simulink model "sample02_speed1"  (R2023a)
settings: Solver=ode1  StartTime=0.0  StopTime=inf  FixedStep=0.005  RelTol=1e-3  EnableMultiTasking=on
libraries: arduinolib x7, simulink x2
settings Model: ExtModeTrigDuration=2  Creator=kawata  LastModifiedBy=kawata
settings SolverCC: AutoInsertRateTranBlk=on
settings DataIOCC: ReturnWorkspaceOutputs=off
settings OptimizationCC: EnhancedBackFolding=on  PassReuseOutputArgsAs=Individual arguments  ZeroExternalMemoryAtStartup=off  ZeroInternalMemoryAtStartup=off  MaxStackSize=64  OptimizeBlockOrder=speed  DifferentSizesBufferReuse=on  OptimizationCustomize=off  EfficientTunableParamExpr=on
settings DebuggingCC: ParameterTunabilityLossMsg=error
settings HardwareCC: ProdBitPerInt=16  ProdBitPerPointer=16  ProdBitPerSizeT=16  ProdBitPerPtrDiffT=16  ProdLargestAtomicFloat=None  ProdWordSize=8  ProdHWDeviceType=Atmel->AVR  UseEmbeddedCoderFeatures=off  UseSimulinkCoderFeatures=off
settings SFSimCC: MATLABDynamicMemAlloc=off
settings RTWCC: Description=Embedded Coder  SystemTargetFile=ert.tlc  HardwareBoard=Arduino Mega 2560  TemplateMakefile=ert_default_tmf  Toolchain=Arduino AVR  BuildConfiguration=Faster Runs  GPUComputeCapability=5.0
settings CodeAppCC: ForceParamTrailComments=on  IgnoreCustomStorageClasses=off  OperatorAnnotations=on  SimulinkDataObjDesc=on  SFDataObjDesc=on  InsertBlockDesc=on
settings ERTTargetCC: SupportContinuousTime=on  SupportNonInlinedSFcns=on  SupportVariableSizeSignals=on  ExtModeTransport=3  ExtModeStaticAlloc=on  ExtModeAutomaticAllocSize=off  ExtModeStaticAllocSize=2048  ExtModeMexFile=ext_xcp  ExtModeIntrfLevel=Level2 - Open

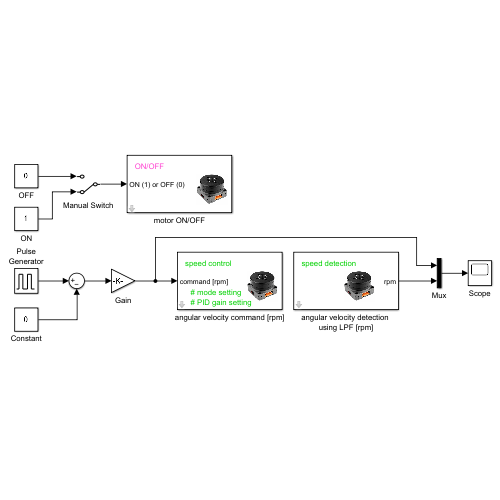
[thumbnail: Simulink's stored preview of the top-level diagram]
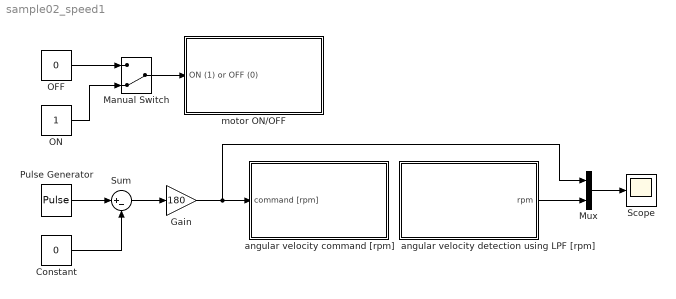
== system sample02_speed1 ==
  Constant : Constant  Value=0
  Gain : Gain  Gain=180
  Manual Switch : ManualSwitch  CurrentSetting=0
  Mux : Mux  Inputs=2
  OFF : Constant  Value=0
  ON : Constant
  Pulse Generator : DiscretePulseGenerator  PulseType=Time based  Period=4  PulseWidth=50  PhaseDelay=1
  Scope : Scope
  Sum : Sum  Inputs=|+-
  angular velocity command [rpm] : Subsystem  mask(angular velocity command [rpm]){I2CAddress=0x64, set_time=0, speed_P=15, speed_I=0.0001, speed_D=400}
      mask prompts: I2CAddress "I2C Address"; set_time "Set Time"; speed_P "P"; speed_I "I"; speed_D "D"
      mask help:
      | speed mode
      | ---------------------------------
      | default value (PID gain of speed controller)
      |  P: 15
      |  I: 0.0001
      |  D: 400
      | ---------------------------------
      | If t ≤ set_time, then PID gain can be set.
      mask DialogControl ParameterGroupVar Prompt: パラメーター
      mask Display:
      | image('roller485.png', [55,10,75,56]);
      | color('green');
      | text(10, 60, 'speed control');
      | text(17, 22, '# mode setting');
      | text(17, 10, '# PID gain setting');
  angular velocity detection using LPF [rpm] : Subsystem  mask{I2CAddress=0x64, sample_time=0.005}
      mask prompts: I2CAddress "I2C Address"; sample_time "Sample Time"
      mask DialogControl ParameterGroupVar Prompt: パラメーター
      mask Display:
      | image('roller485.png', [30,10,75,56]);
      | color('green');
      | text(10, 60, 'speed detection');
  motor ON/OFF : Subsystem  mask{I2CAddress=0x64}
      mask prompts: I2CAddress "I2C Address"
      mask help:
      | 0: motor off
      | 1: motor on
      mask DialogControl ParameterGroupVar Prompt: パラメーター
      mask Display:
      | image('roller485.png', [55,10,75,56]);
      | color('magenta');
      | text(10, 60, 'ON/OFF');
  wires:
  Manual Switch/1 -> motor ON/OFF/1(ON (1) or OFF (0))
  OFF/1 -> Manual Switch/1
  ON/1 -> Manual Switch/2
  Gain/1 -> angular velocity command [rpm]/1(command [rpm]), Mux/1
  Sum/1 -> Gain/1
  Constant/1 -> Sum/2
  Pulse Generator/1 -> Sum/1
  angular velocity detection using LPF [rpm]/1(rpm) -> Mux/2
  Mux/1 -> Scope/1

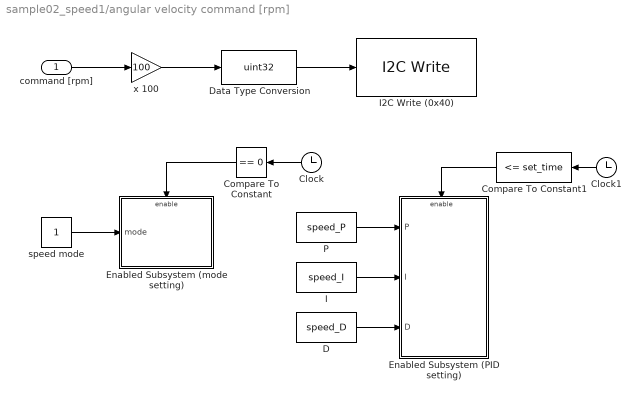
== system sample02_speed1/angular velocity command [rpm] ==
  command [rpm] : Inport
  "Clock " : Clock
  Clock1 : Clock
  Compare To Constant : simulink/Logic and Bit Operations/Compare To Constant  relop===  const=0  OutDataTypeStr=boolean
  Compare To Constant1 : simulink/Logic and Bit Operations/Compare To Constant  relop=<=  const=set_time  OutDataTypeStr=boolean
  D : Constant  Value=speed_D
  Data Type Conversion : DataTypeConversion  OutDataTypeStr=uint32  SaturateOnIntegerOverflow=off  RndMeth=Floor
  Enabled Subsystem (PID setting) : Subsystem  TreatAsAtomicUnit=on
  Enabled Subsystem (mode setting) : Subsystem  TreatAsAtomicUnit=on
  I : Constant  Value=speed_I
  I2C Write (0x40) : arduinolib/I2C Write  I2CModule=0  Mode=Master  SlaveAddress=I2CAddress  SlaveByteOrder=LittleEndian  Direction=Transmitter  RegisterAddressMode=on  RegisterAddress=0x40  SlaveDataType=uint8  DataLength=1  NoAck=off  RepeatedStart=off  OutputStatus=off  blockPlatform=ARDUINO
  P : Constant  Value=speed_P
  speed mode : Constant
  x 100 : Gain  Gain=100
  wires:
  x 100/1 -> Data Type Conversion/1
  command [rpm]/1 -> x 100/1
  Data Type Conversion/1 -> I2C Write (0x40)/1
  I/1 -> Enabled Subsystem (PID setting)/2(I)
  Clock1/1 -> Compare To Constant1/1
  P/1 -> Enabled Subsystem (PID setting)/1(P)
  speed mode/1 -> Enabled Subsystem (mode setting)/1(mode)
  Compare To Constant1/1 -> Enabled Subsystem (PID setting)/Enable
  Compare To Constant/1 -> Enabled Subsystem (mode setting)/Enable
  "Clock "/1 -> Compare To Constant/1
  D/1 -> Enabled Subsystem (PID setting)/3(D)

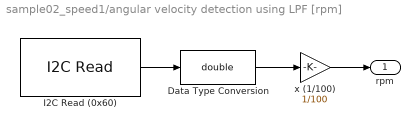
== system sample02_speed1/angular velocity detection using LPF [rpm] ==
  Data Type Conversion : DataTypeConversion  OutDataTypeStr=double  SaturateOnIntegerOverflow=off  RndMeth=Floor
  I2C Read (0x60) : arduinolib/I2C Read  I2CModule=0  Mode=Master  SlaveAddress=0x64  SlaveByteOrder=LittleEndian  Direction=Receiver  RegisterAddressMode=on  RegisterAddress=0x60  SlaveDataType=int32  DataLength=1  NoAck=off  RepeatedStart=off  OutputStatus=off  blockPlatform=ARDUINO  SampleTime=sample_time
  x (1/100) : Gain  Gain=1/100
  rpm : Outport
  wires:
  I2C Read (0x60)/1 -> Data Type Conversion/1
  Data Type Conversion/1 -> x (1/100)/1
  x (1/100)/1 -> rpm/1

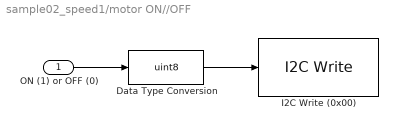
== system sample02_speed1/motor ON//OFF ==
  ON (1) or OFF (0) : Inport
  Data Type Conversion : DataTypeConversion  OutDataTypeStr=uint8  SaturateOnIntegerOverflow=off  RndMeth=Floor
  I2C Write (0x00) : arduinolib/I2C Write  I2CModule=0  Mode=Master  SlaveAddress=I2CAddress  SlaveByteOrder=BigEndian  Direction=Transmitter  RegisterAddressMode=on  RegisterAddress=0x00  SlaveDataType=uint8  DataLength=1  NoAck=off  RepeatedStart=off  OutputStatus=off  blockPlatform=ARDUINO
  wires:
  Data Type Conversion/1 -> I2C Write (0x00)/1
  ON (1) or OFF (0)/1 -> Data Type Conversion/1

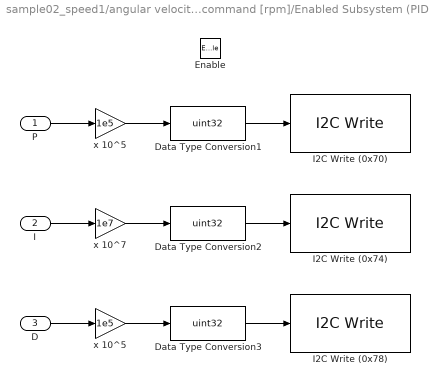
== system sample02_speed1/angular velocity command [rpm]/Enabled Subsystem (PID setting) ==
  P : Inport
  I : Inport  Port=2
  D : Inport  Port=3
  Enable : EnablePort
  " x 10^5 " : Gain  Gain=1e5
  Data Type Conversion1 : DataTypeConversion  OutDataTypeStr=uint32  SaturateOnIntegerOverflow=off  RndMeth=Floor
  Data Type Conversion2 : DataTypeConversion  OutDataTypeStr=uint32  SaturateOnIntegerOverflow=off  RndMeth=Floor
  Data Type Conversion3 : DataTypeConversion  OutDataTypeStr=uint32  SaturateOnIntegerOverflow=off  RndMeth=Floor
  I2C Write (0x70) : arduinolib/I2C Write  I2CModule=0  Mode=Master  SlaveAddress=I2CAddress  SlaveByteOrder=LittleEndian  Direction=Transmitter  RegisterAddressMode=on  RegisterAddress=0x70  SlaveDataType=uint8  DataLength=1  NoAck=off  RepeatedStart=off  OutputStatus=off  blockPlatform=ARDUINO
  I2C Write (0x74) : arduinolib/I2C Write  I2CModule=0  Mode=Master  SlaveAddress=I2CAddress  SlaveByteOrder=LittleEndian  Direction=Transmitter  RegisterAddressMode=on  RegisterAddress=0x74  SlaveDataType=uint8  DataLength=1  NoAck=off  RepeatedStart=off  OutputStatus=off  blockPlatform=ARDUINO
  I2C Write (0x78) : arduinolib/I2C Write  I2CModule=0  Mode=Master  SlaveAddress=I2CAddress  SlaveByteOrder=LittleEndian  Direction=Transmitter  RegisterAddressMode=on  RegisterAddress=0x78  SlaveDataType=uint8  DataLength=1  NoAck=off  RepeatedStart=off  OutputStatus=off  blockPlatform=ARDUINO
  x 10^5 : Gain  Gain=1e5
  x 10^7 : Gain  Gain=1e7
  wires:
  " x 10^5 "/1 -> Data Type Conversion3/1
  x 10^7/1 -> Data Type Conversion2/1
  x 10^5/1 -> Data Type Conversion1/1
  Data Type Conversion1/1 -> I2C Write (0x70)/1
  Data Type Conversion3/1 -> I2C Write (0x78)/1
  Data Type Conversion2/1 -> I2C Write (0x74)/1
  D/1 -> " x 10^5 "/1
  I/1 -> x 10^7/1
  P/1 -> x 10^5/1

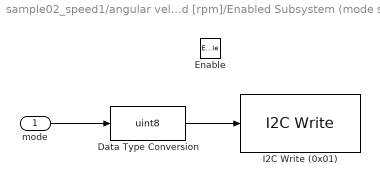
== system sample02_speed1/angular velocity command [rpm]/Enabled Subsystem (mode setting) ==
  mode : Inport
  Enable : EnablePort
  Data Type Conversion : DataTypeConversion  OutDataTypeStr=uint8  SaturateOnIntegerOverflow=off  RndMeth=Floor
  I2C Write (0x01) : arduinolib/I2C Write  I2CModule=0  Mode=Master  SlaveAddress=I2CAddress  SlaveByteOrder=BigEndian  Direction=Transmitter  RegisterAddressMode=on  RegisterAddress=0x01  SlaveDataType=uint8  DataLength=1  NoAck=off  RepeatedStart=off  OutputStatus=off  blockPlatform=ARDUINO
  wires:
  Data Type Conversion/1 -> I2C Write (0x01)/1
  mode/1 -> Data Type Conversion/1
